simulink model "helicopter"  (R2014b)
settings: Solver=ode45  StartTime=0.0  StopTime=10.0  RelTol=1e-3
undefined symbols (not defined in the file): a, i, K
settings Model: Creator=alex  LastModifiedBy=alex
settings DebuggingCC: SolverPrmCheckMsg=none

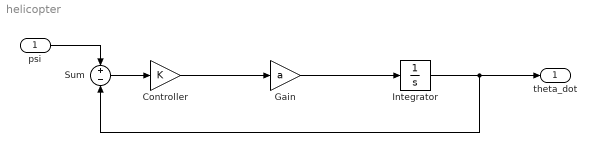
== system helicopter ==
  psi : Inport
  "Controller " : Gain  Gain=K
  Gain : Gain  Gain=a
  Integrator : Integrator  InitialCondition=i
  Sum : Sum  Inputs=+-
  theta_dot : Outport
  wires:
  Gain/1 -> Integrator/1
  Integrator/1 -> Sum/2, theta_dot/1
  "Controller "/1 -> Gain/1
  psi/1 -> Sum/1
  Sum/1 -> "Controller "/1
